simulink model "experimentSim_2018a"  (R2018a)
settings: Solver=FixedStepDiscrete  StartTime=0.0  StopTime=Inf  FixedStep=0.0004  RelTol=1e-3  EnableMultiTasking=on
values from neighbouring files (symbols this model uses):
  haptic_setup = HapticSetup(config)    [experiment.m]
undefined symbols (not defined in the file or in its folder): config, National_Instruments, PCI, PCIe
libraries: sldrtlib x3, dspsigops x1, simulink x1, dspstat3 x1
settings Model: SimulationMode=external  ExtModeTrigDuration=5000000  Creator=omer  LastModifiedBy=omer
settings DataIOCC: MaxDataPoints=10000000  SaveFormat=Array
settings DebuggingCC: SolverPrmCheckMsg=warning  SFUnexpectedBacktrackingDiag=warning  SFNoUnconditionalDefaultTransitionDiag=warning  SFExecutionAtInitializationDiag=none
settings ModelReferenceCC: PropagateSignalLabelsOutOfModel=off
settings RTWCC: SystemTargetFile=sldrt.tlc  TemplateMakefile=sldrt.tmf  Description=Simulink Desktop Real-Time  RTWCompilerOptimization=on
settings CodeAppCC: MaxIdLength=95  StateflowObjectComments=on
settings SimulinkDesktopRealTimeCC: TargetPreCompLibLocation=C:\Program Files\MATLAB\R2018a\toolbox\sldrt\lib\win64  TargetLangStandard=C89/C90 (ANSI)  SupportVariableSizeSignals=off
settings ConfigComp: CovMetricSettings=dw  CovSaveCumulativeToWorkspaceVar=on  CovSaveSingleToWorkspaceVar=on  CovExternalEMLEnable=off  CovSFcnEnable=off

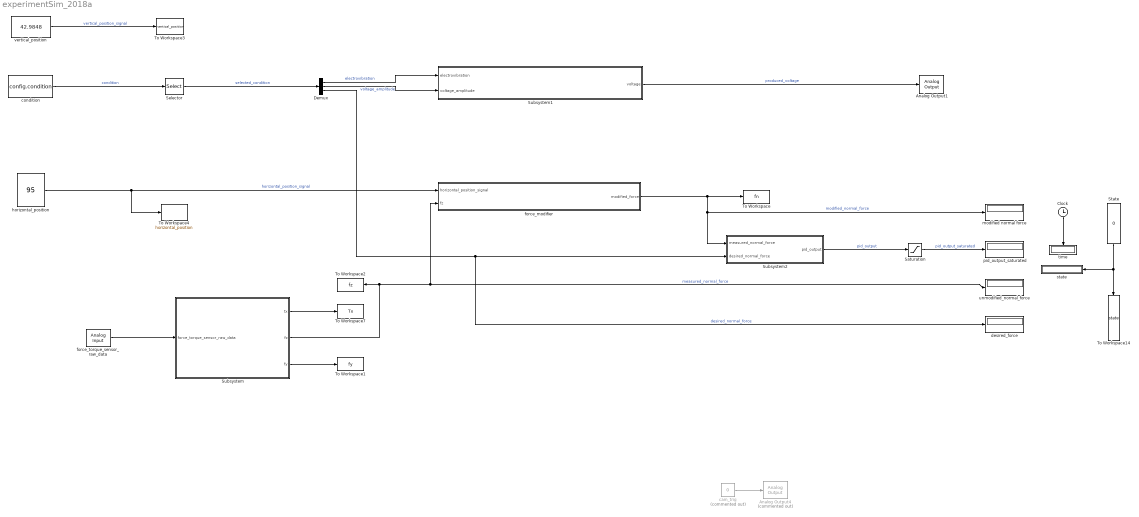
== system experimentSim_2018a ==
  Analog Output1 : sldrtlib/Analog Output  SampleTime=0.0004  MaxMissedTicks=10  ShowMissedTicks=off  YieldWhenWaiting=off  DrvName=National_Instruments/PCIe-6321  DrvAddress=4294967295  DrvOptions=[0 0 0 0 0 0 0]  Channels=1  RangeMode=1  VoltRange=1  InitialValue=0  FinalValue=0
      settings: AttributesFormatString=National Instruments\nPCIe-6321 [auto]
  Analog Output4 : sldrtlib/Analog Output  Commented=on  SampleTime=0.0004  MaxMissedTicks=10  ShowMissedTicks=off  YieldWhenWaiting=off  DrvName=National_Instruments/PCIe-6321  DrvAddress=4294967295  DrvOptions=[0 255 65535 0 0 0 0]  Channels=2  RangeMode=1  VoltRange=1  InitialValue=0  FinalValue=0
      settings: AttributesFormatString=National Instruments\nPCIe-6321 [auto]
  Clock : Clock
  Demux : Demux  Outputs=3
  Saturation : Saturate  UpperLimit=50  LowerLimit=-50
  Selector : Selector  NumberOfDimensions=2  InputPortWidth=3  IndexOptions=Index vector (dialog),Select all  Indices=[haptic_setup.current_sliding_iteration],haptic_setup.config.current_sliding_iteration  OutputSizes=1,1
  State : Constant  Value=0
  Subsystem : Subsystem
  Subsystem1 : Subsystem
  Subsystem2 : Subsystem
  To Workspace : ToWorkspace  VariableName=fn  SaveFormat=Structure With Time  SampleTime=-1
  To Workspace1 : ToWorkspace  VariableName=fy  SaveFormat=Structure With Time  SampleTime=-1
  To Workspace14 : ToWorkspace  VariableName=state  SaveFormat=Structure With Time  SampleTime=-1
  To Workspace2 : ToWorkspace  VariableName=fz  SaveFormat=Structure With Time  SampleTime=-1
  To Workspace3 : ToWorkspace  VariableName=vertical_position  SaveFormat=Structure With Time  SampleTime=-1
  To Workspace4 : ToWorkspace  VariableName=horizontal_position  SaveFormat=Structure With Time  SampleTime=-1
  To Workspace7 : ToWorkspace  VariableName=Tx  SaveFormat=Structure With Time  SampleTime=-1
  cam_trig : Constant  Commented=on  Value=0
  condition : Constant  Value=config.condition  VectorParams1D=off
  desired_force : Display
  force_modifier : Subsystem
  force_torque_sensor_raw_data : sldrtlib/Analog Input  SampleTime=0.0004  MaxMissedTicks=10  ShowMissedTicks=off  YieldWhenWaiting=off  DrvName=National_Instruments/PCI-6034E  DrvAddress=4294967295  DrvOptions=[0 0 0 0 0 0]  Channels=1:6  RangeMode=1  VoltRange=1  DataType=1
      settings: AttributesFormatString=National Instruments\nPCI-6034E [auto]
  horizontal_position : Constant  Value=95
  modified normal force : Display
  pid_output_saturated : Display
  state : Display
  "time " : Display
  unmodified_normal_force : Display
  vertical_position : Constant  Value=42.9848
  wires:
  force_modifier/1(modified_force) -> To Workspace/1, Subsystem2/1(measured_normal_force), modified normal force/1  "modified_normal_force"
  Saturation/1 -> pid_output_saturated/1  "pid_output_saturated"
  cam_trig/1 -> Analog Output4/1
  condition/1 -> Selector/1  "condition"
  Demux/3 -> desired_force/1, Subsystem2/2(desired_normal_force)  "desired_normal_force"
  vertical_position/1 -> To Workspace3/1  "vertical_position_signal"
  State/1 -> state/1, To Workspace14/1
  Selector/1 -> Demux/1  "selected_condition"
  Subsystem/2(fz) -> unmodified_normal_force/1, force_modifier/2(fz), To Workspace2/1  "measured_normal_force"
  force_torque_sensor_raw_data/1 -> Subsystem/1(force_torque_sensor_raw_data)
  Subsystem/1(tx) -> To Workspace7/1
  Subsystem/3(fy) -> To Workspace1/1
  Demux/1 -> Subsystem1/1(electrovibration)  "electrovibration"
  Demux/2 -> Subsystem1/2(voltage_amplitude)  "voltage_amplitude"
  Subsystem1/1(voltage) -> Analog Output1/1  "produced_voltage"
  horizontal_position/1 -> To Workspace4/1, force_modifier/1(horizontal_position_signal)  "horizontal_position_signal"
  Subsystem2/1(pid_output) -> Saturation/1  "pid_output"
  Clock/1 -> "time "/1

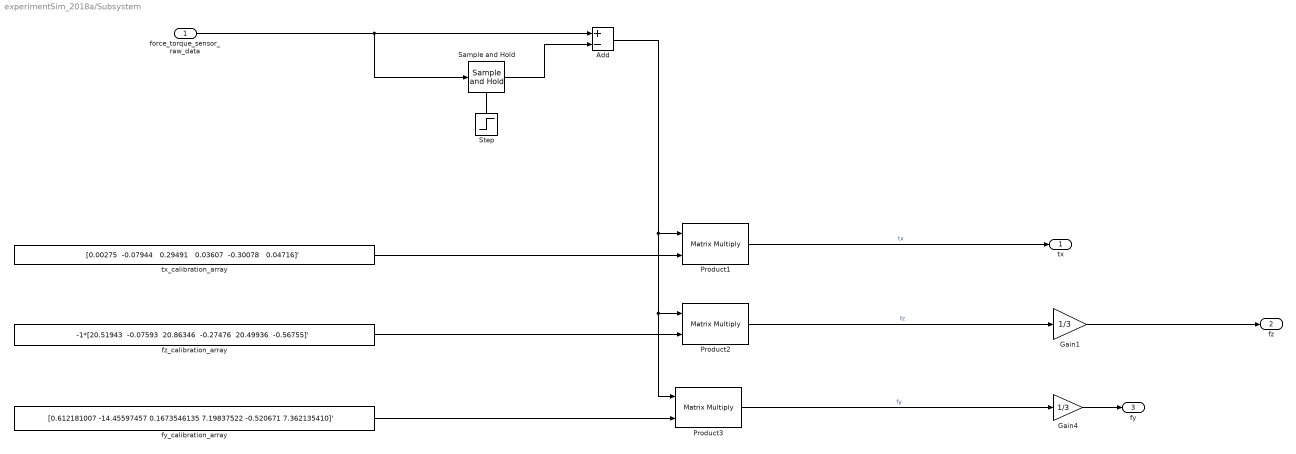
== system experimentSim_2018a/Subsystem ==
  force_torque_sensor_raw_data : Inport
  Add : Sum  Inputs=+-
  Gain1 : Gain  Gain=1/3
  Gain4 : Gain  Gain=1/3
  Product1 : Product  Multiplication=Matrix(*)
  Product2 : Product  Multiplication=Matrix(*)
  Product3 : Product  Multiplication=Matrix(*)
  Sample and Hold : dspsigops/Sample and Hold  trig=Rising edge  initCond=0  latchinput=off
  Step : Step  Time=0.3  SampleTime=0
  fy_calibration_array : Constant  Value=[0.612181007 -14.45597457 0.1673546135 7.19837522 -0.520671 7.362135410]'
  fz_calibration_array : Constant  Value="-1*[20.51943  -0.07593  20.86346  -0.27476  20.49936  -0.56755]'"
  tx_calibration_array : Constant  Value="[0.00275  -0.07944   0.29491   0.03607  -0.30078   0.04716]'"
  tx : Outport  VectorParamsAs1DForOutWhenUnconnected=on
  fz : Outport  Port=2  VectorParamsAs1DForOutWhenUnconnected=on
  fy : Outport  Port=3  VectorParamsAs1DForOutWhenUnconnected=on
  wires:
  Gain4/1 -> fy/1
  Sample and Hold/1 -> Add/2
  Step/1 -> Sample and Hold/Trigger
  Add/1 -> Product1/1, Product2/1, Product3/1
  Product3/1 -> Gain4/1  "fy"
  tx_calibration_array/1 -> Product1/2
  fy_calibration_array/1 -> Product3/2
  Gain1/1 -> fz/1
  fz_calibration_array/1 -> Product2/2
  force_torque_sensor_raw_data/1 -> Add/1, Sample and Hold/1
  Product1/1 -> tx/1  "tx"
  Product2/1 -> Gain1/1  "fz"

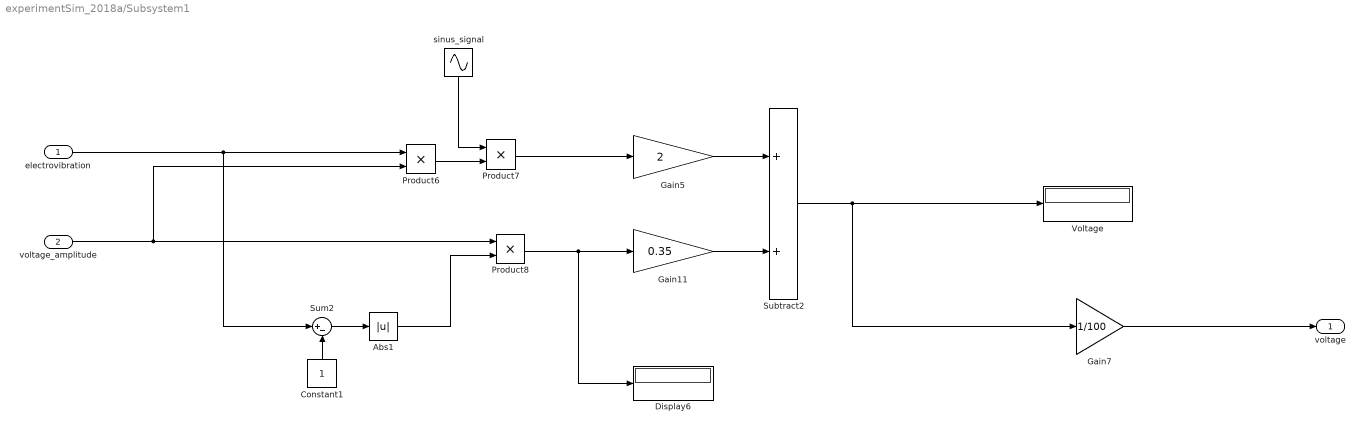
== system experimentSim_2018a/Subsystem1 ==
  electrovibration : Inport
  voltage_amplitude : Inport  Port=2
  Abs1 : Abs
  Constant1 : Constant
  Display6 : Display
  Gain11 : Gain  Gain=0.35
  Gain5 : Gain  Gain=2
  Gain7 : Gain  Gain=1/100
  Product6 : Product
  Product7 : Product
  Product8 : Product
  Subtract2 : Sum
  Sum2 : Sum  Inputs=|+-
  Voltage : Display
  sinus_signal : Sin  Frequency=2*pi*125  Samples=1000  SampleTime=0
  voltage : Outport  VectorParamsAs1DForOutWhenUnconnected=on
  wires:
  Product7/1 -> Gain5/1
  Gain11/1 -> Subtract2/2
  Product8/1 -> Display6/1, Gain11/1
  Gain5/1 -> Subtract2/1
  sinus_signal/1 -> Product7/1
  electrovibration/1 -> Product6/1, Sum2/1
  voltage_amplitude/1 -> Product8/1, Product6/2
  Constant1/1 -> Sum2/2
  Gain7/1 -> voltage/1
  Sum2/1 -> Abs1/1
  Product6/1 -> Product7/2
  Subtract2/1 -> Gain7/1, Voltage/1
  Abs1/1 -> Product8/2

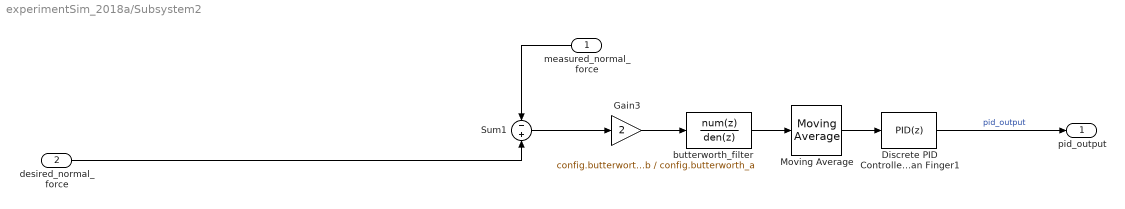
== system experimentSim_2018a/Subsystem2 ==
  measured_normal_force : Inport
  desired_normal_force : Inport  Port=2
  Discrete PID Controller Human Finger1 : simulink/Continuous/PID Controller  Controller=PID  TimeDomain=Discrete-time  SampleTime=-1  IntegratorMethod=Forward Euler  FilterMethod=Forward Euler  Form=Parallel  UseFilter=on  ControllerParametersSource=internal  P=9*.33*1.8  I=2/(.87*1.8)  D=(.87*1.4)/3  N=3  InitialConditionSource=internal  InitialConditionForIntegrator=0  InitialConditionForFilter=0  ExternalReset=none  LimitOutput=off  UpperSaturationLimit=inf  LowerSaturationLimit=-inf  LinearizeAsGain=off  AntiWindupMode=none  Kb=1  TrackingMode=off  Kt=1  PParamMin=[]  PParamMax=[]  IParamMin=[]  IParamMax=[]  DParamMin=[]  DParamMax=[]  NParamMin=[]  NParamMax=[]  KbParamMin=[]  KbParamMax=[]  KtParamMin=[]  KtParamMax=[]  POutMin=[]  POutMax=[]  IOutMin=[]  IOutMax=[]  DOutMin=[]  DOutMax=[]  NOutMin=[]  NOutMax=[]  KbOutMin=[]  KbOutMax=[]  KtOutMin=[]  KtOutMax=[]  IntegratorOutMin=[]  IntegratorOutMax=[]  FilterOutMin=[]  FilterOutMax=[]  SumOutMin=[]  SumOutMax=[]  SumI1OutMin=[]  SumI1OutMax=[]  SumI2OutMin=[]  SumI2OutMax=[]  SumI3OutMin=[]  SumI3OutMax=[]  SumDOutMin=[]  SumDOutMax=[]  SaturationOutMin=[]  SaturationOutMax=[]  IntegratorContinuousStateAttributes=''  IntegratorStateMustResolveToSignalObject=off  IntegratorRTWStateStorageClass=Auto  FilterContinuousStateAttributes=''  FilterStateMustResolveToSignalObject=off  FilterRTWStateStorageClass=Auto  DifferentiatorICPrevScaledInput=0  DifferentiatorOutMin=[]  DifferentiatorOutMax=[]  FilterDiffOutCoefMin=[]  FilterDiffOutCoefMax=[]  SumDenOutMin=[]  SumDenOutMax=[]  SumNumOutMin=[]  SumNumOutMax=[]  ReciprocalOutMin=[]  ReciprocalOutMax=[]  DivideOutMin=[]  DivideOutMax=[]  TunerSelectOption=Transfer Function Based (PID Tuner App)
  Gain3 : Gain  Gain=2
  Moving Average : dspstat3/Moving Average  Method=Sliding window  ForgettingFactorPort=off  SpecifyWindowLength=on  WindowLength=50  ForgettingFactor=0.9  SimulateUsing=Code generation
  Sum1 : Sum  Inputs=-+
  butterworth_filter : DiscreteFilter  Numerator=config.butterworth_b  Denominator=config.butterworth_a
  pid_output : Outport  VectorParamsAs1DForOutWhenUnconnected=on
  wires:
  Sum1/1 -> Gain3/1
  butterworth_filter/1 -> Moving Average/1
  Moving Average/1 -> Discrete PID Controller Human Finger1/1
  desired_normal_force/1 -> Sum1/2
  Discrete PID Controller Human Finger1/1 -> pid_output/1  "pid_output"
  Gain3/1 -> butterworth_filter/1
  measured_normal_force/1 -> Sum1/1

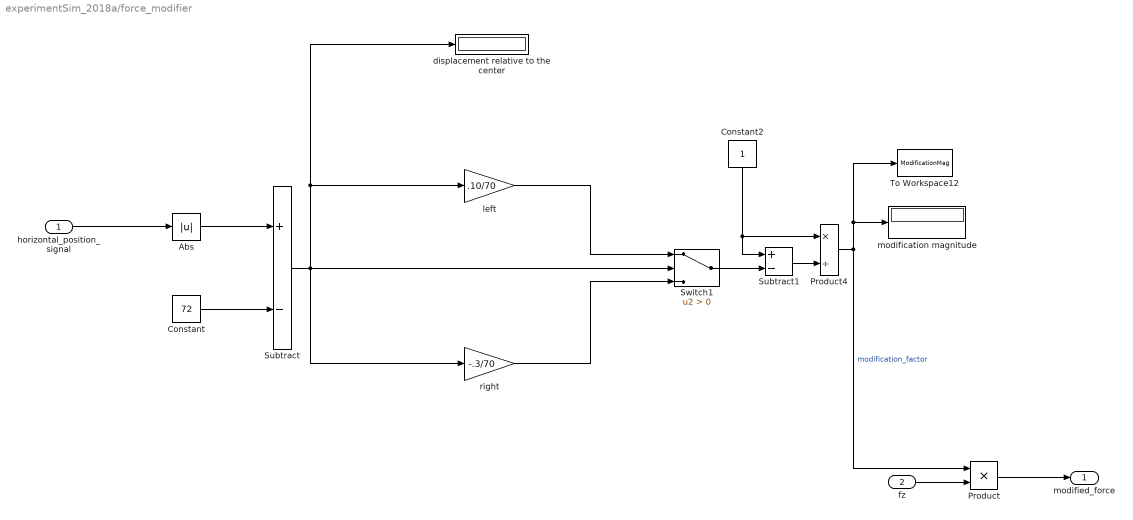
== system experimentSim_2018a/force_modifier ==
  horizontal_position_signal : Inport
  fz : Inport  Port=2
  " displacement relative to the center" : Display
  Abs : Abs
  Constant : Constant  Value=72
  Constant2 : Constant
  Product : Product
  Product4 : Product  Inputs=*/
  Subtract : Sum  Inputs=+-
  Subtract1 : Sum  Inputs=+-
  Switch1 : Switch  Criteria=u2 > Threshold
  To Workspace12 : ToWorkspace  VariableName=ModificationMag  SaveFormat=Structure With Time  SampleTime=-1
  left : Gain  Gain=.10/70
  modification magnitude : Display
  right : Gain  Gain=-.3/70
  modified_force : Outport  VectorParamsAs1DForOutWhenUnconnected=on
  wires:
  Switch1/1 -> Subtract1/2
  Abs/1 -> Subtract/1
  Constant2/1 -> Product4/1, Subtract1/1
  left/1 -> Switch1/1
  Product4/1 -> Product/1, To Workspace12/1, modification magnitude/1  "modification_factor"
  horizontal_position_signal/1 -> Abs/1
  Constant/1 -> Subtract/2
  Subtract1/1 -> Product4/2
  Subtract/1 -> " displacement relative to the center"/1, left/1, Switch1/2, right/1
  right/1 -> Switch1/3
  fz/1 -> Product/2
  Product/1 -> modified_force/1
